simulink model "clase24112020"  (R2020b)
settings: Solver=VariableStepAuto  StartTime=0.0  StopTime=inf  RelTol=1e-3
libraries: dspvision x3, dsparch4 x1, commanapbnd3 x1
settings Model: Creator=fer-1  LastModifiedBy=fer-1

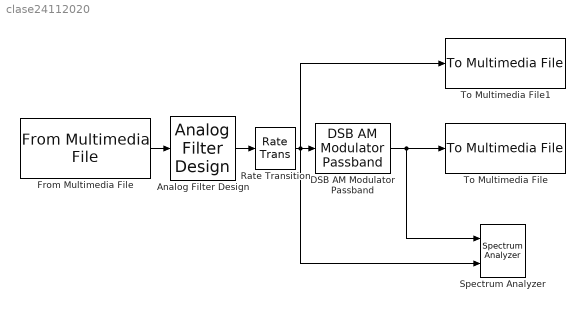
== system clase24112020 ==
  Analog Filter Design : dsparch4/Analog Filter Design  method=Butterworth  filttype=Lowpass  N=8  Wlo=2*pi*4e3  Whi=80  Rp=2  Rs=40
  DSB AM Modulator Passband : commanapbnd3/DSB AM Modulator Passband  Fc=10e3  Ph=0  Offset=1
      settings: SourceProductBaseCode=CM
  From Multimedia File : dspvision/From Multimedia File  inputFilename=speech_dft.mp3  readRange=[1 Inf]  loop=on  numPlays=inf  outputStreams=Audio only  videoDataType=single  audioDataType=double  inheritSampleTime=on  userDefinedSampleTime=1/30  noAudioOutput=off  isIntensityVideo=off  fourcc=RGB  colorVideoFormat=Separate color signals  outputEOF=off  dataOrg=Column-major  audioFrameSize=1  computeAudioFrameSize=off  outSamplingMode=Sample based
  Rate Transition : RateTransition  OutPortSampleTime=1/44100/2
  Spectrum Analyzer : SpectrumAnalyzer  NumInputPorts=2
  To Multimedia File : dspvision/To Multimedia File  outputFilename=Salida_mod.wav  streamSelection=Audio only  videoCompressor=None (uncompressed)  audioCompressor=None (uncompressed)  imagePorts=Separate color signals  fileType=WAV  audioDatatype=16-bit integer  fourcc=RGB  videoQuality=75  mj2000CompFactor=10
  To Multimedia File1 : dspvision/To Multimedia File  outputFilename=SalidaFiltro.wav  streamSelection=Audio only  videoCompressor=None (uncompressed)  audioCompressor=None (uncompressed)  imagePorts=Separate color signals  fileType=WAV  audioDatatype=16-bit integer  fourcc=RGB  videoQuality=75  mj2000CompFactor=10
  wires:
  From Multimedia File/1 -> Analog Filter Design/1
  Analog Filter Design/1 -> Rate Transition/1
  DSB AM Modulator Passband/1 -> Spectrum Analyzer/1, To Multimedia File/1
  Rate Transition/1 -> Spectrum Analyzer/2, To Multimedia File1/1, DSB AM Modulator Passband/1
